simulink model "generalizedPlantDistwoF_unc"  (R2019a)
settings: Solver=VariableStepAuto  StartTime=0.0  StopTime=10.0  RelTol=1e-3  EnableMultiTasking=on
undefined symbols (not defined in the file): np, nq, nu, ny, nzKS, nzS
libraries: cstblocks x1
settings Model: Creator=chris  LastModifiedBy=Marlin Siebert
settings DataIOCC: ReturnWorkspaceOutputs=off
settings OptimizationCC: LifeSpan=inf
settings DebuggingCC: SFUnexpectedBacktrackingDiag=warning  SFNoUnconditionalDefaultTransitionDiag=warning  SFExecutionAtInitializationDiag=none  ArithmeticOperatorsInVariantConditions=warning
settings SFSimCC: SimUseLocalCustomCode=off
settings RTWCC: RTWUseLocalCustomCode=off
settings CodeAppCC: StateflowObjectComments=on
settings GRTTargetCC: TargetLangStandard=C89/C90 (ANSI)  GeneratePreprocessorConditionals=Disable all
settings ConfigComp: CovMetricSettings=dw  CovHtmlReporting=on  CovSaveCumulativeToWorkspaceVar=on  CovSaveSingleToWorkspaceVar=on  CovExternalEMLEnable=off

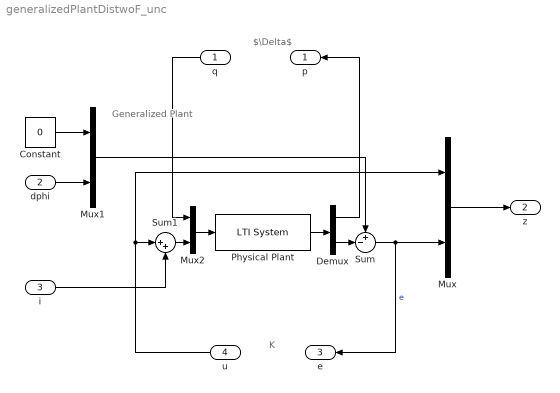
== system generalizedPlantDistwoF_unc ==
  note: K
  note: Generalized Plant
  note: $\Delta$
  q : Inport
  dphi : Inport  Port=2
  i : Inport  Port=3
  u : Inport  Port=4
  Constant : Constant  Value=0
  Demux : Demux  Outputs=[np, ny]
  Mux : Mux  Inputs=[nzKS, nzS]
  Mux1 : Mux  Inputs=2
  Mux2 : Mux  Inputs=[nq, nu]
  Physical Plant : cstblocks/LTI System  sys=G_gen_cert  IC=[]
  Sum : Sum  Inputs=+-|
  Sum1 : Sum  Inputs=|++
  p : Outport
  z : Outport  Port=2
  e : Outport  Port=3
  wires:
  Demux/2 -> Sum/2
  Sum/1 -> Mux/2, e/1  "e"
  Mux/1 -> z/1
  Constant/1 -> Mux1/1
  dphi/1 -> Mux1/2
  Mux1/1 -> Sum/1
  i/1 -> Sum1/2
  u/1 -> Mux/1, Sum1/1
  Sum1/1 -> Mux2/2
  q/1 -> Mux2/1
  Demux/1 -> p/1
  Physical Plant/1 -> Demux/1
  Mux2/1 -> Physical Plant/1
